simulink model "ASI_switch_Sami_FAHIM_R2022a"  (R2022a)
settings: Solver=VariableStepAuto  StartTime=0.0  StopTime=0.04  RelTol=1e-3
undefined symbols (not defined in the file): Az_I, Bz_I, Cz_I, Fz_I, Gz_I, Te, Vd
libraries: spsIGBTDiodeLib x4, cstblocks x4, spsSeriesRLCBranchLib x3, spsCurrentMeasurementLib x1, spsDCVoltageSourceLib x1, spsVoltageMeasurementLib x1, spspowerguiLib x1, simulink x1
settings Model: Creator=xshi  LastModifiedBy=sfahim

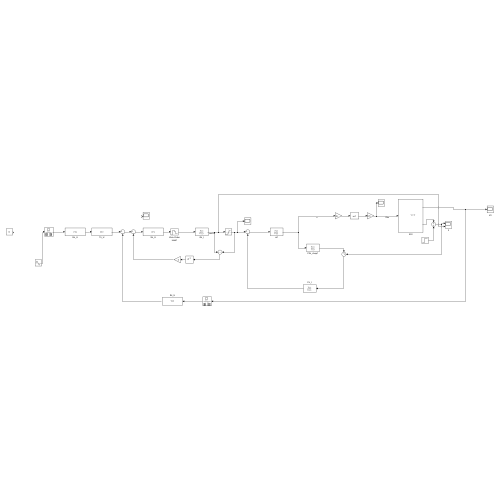
[thumbnail: Simulink's stored preview of the top-level diagram]
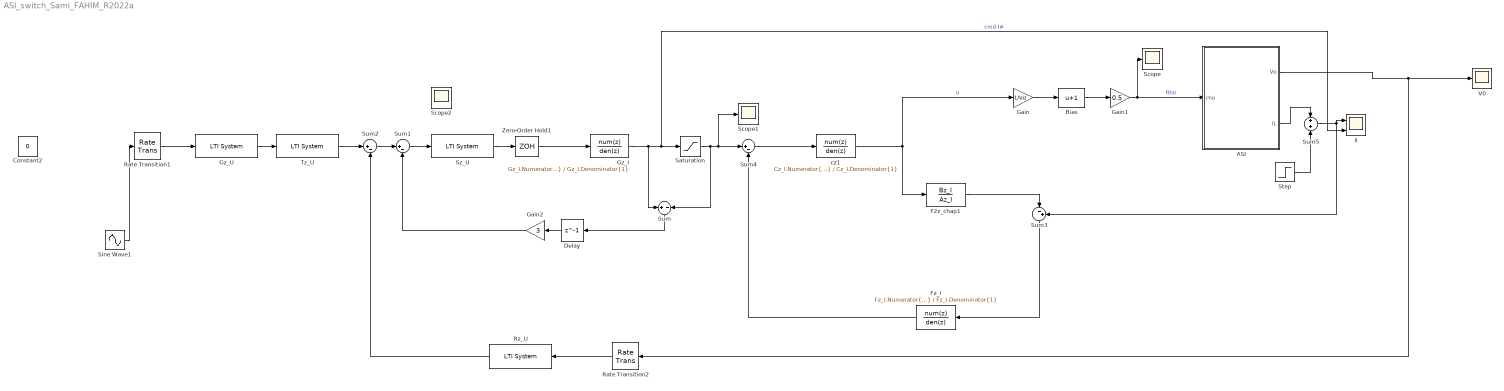
== system ASI_switch_Sami_FAHIM_R2022a ==
  ASI : Subsystem
      mask Display: image('C:\Users\xshi\Documents\Xuefang\Enseignement\4GE\COURS4GE\DS\DS 2024\Semestre 1\Matlab\ASI.png'); % Use "Edit Image" on toolstrip to change.
  Bias : Bias  Bias=1  SaturateOnIntegerOverflow=off
  Constant2 : Constant  Value=0  SampleTime=Te
  Delay : Delay  DelayLength=1
  F2z_chap1 : DiscreteTransferFcn  Numerator=Bz_I  Denominator=Az_I  SampleTime=Te
  Fz_I : DiscreteTransferFcn  Numerator=Fz_I.Numerator{1}  Denominator=Fz_I.Denominator{1}  SampleTime=Te
  Gain : Gain  Gain=1/Vd
  Gain1 : Gain  Gain=0.5
  Gain2 : Gain  Gain=3
  Gz_I : DiscreteTransferFcn  Numerator=Gz_I.Numerator{1}  Denominator=Gz_I.Denominator{1}  SampleTime=Te
  Gz_U : cstblocks/LTI System  sys=Gz_U  IC=[]
  Il : Scope  NumInputPorts=2
  Rate Transition1 : RateTransition  OutPortSampleTime=Te
  Rate Transition2 : RateTransition  OutPortSampleTime=Te
  Rz_U : cstblocks/LTI System  sys=Rz_U  IC=[]
  Saturation : Saturate  UpperLimit=25  LowerLimit=-25
  Scope : Scope
  Scope1 : Scope
  Scope2 : Scope
  Sine Wave1 : Sin  Amplitude=230  Frequency=314  SampleTime=0
  Step : Step  Time=0.01  After=0  SampleTime=0
  Sum : Sum  Inputs=+|-
  Sum1 : Sum  Inputs=|+-
  Sum2 : Sum  Inputs=|+-
  Sum3 : Sum  Inputs=|-+
  Sum4 : Sum  Inputs=|+-
  Sum5 : Sum  Inputs=+|+
  Sz_U : cstblocks/LTI System  sys=Sz_U  IC=[]
  Tz_U : cstblocks/LTI System  sys=Tz_U  IC=[]
  V0 : Scope
  Zero-Order Hold1 : ZeroOrderHold  SampleTime=Te
  cz1 : DiscreteTransferFcn  Numerator=Cz_I.Numerator{1}  Denominator=Cz_I.Denominator{1}  SampleTime=Te
  wires:
  Gain/1 -> Bias/1
  ASI/1(Vo) -> Rate Transition2/1, V0/1
  ASI/2(IL) -> Sum5/1
  Sz_U/1 -> Zero-Order Hold1/1
  Gz_U/1 -> Tz_U/1
  Rate Transition2/1 -> Rz_U/1
  Tz_U/1 -> Sum2/1
  Rz_U/1 -> Sum2/2
  Rate Transition1/1 -> Gz_U/1
  Sum3/1 -> Fz_I/1
  cz1/1 -> Gain/1, F2z_chap1/1  "u"
  Fz_I/1 -> Sum4/2
  Sum4/1 -> cz1/1
  Gz_I/1 -> Sum/1, Il/2, Saturation/1  "cmd I#"
  Zero-Order Hold1/1 -> Gz_I/1
  F2z_chap1/1 -> Sum3/1
  Bias/1 -> Gain1/1
  Gain1/1 -> Scope/1, ASI/1(rho)  "Rho"
  Sum/1 -> Delay/1
  Sum5/1 -> Sum3/2, Il/1
  Step/1 -> Sum5/2
  Delay/1 -> Gain2/1
  Saturation/1 -> Sum/2, Scope1/1, Sum4/1
  Sum2/1 -> Sum1/1
  Gain2/1 -> Sum1/2
  Sum1/1 -> Sz_U/1
  Sine Wave1/1 -> Rate Transition1/1

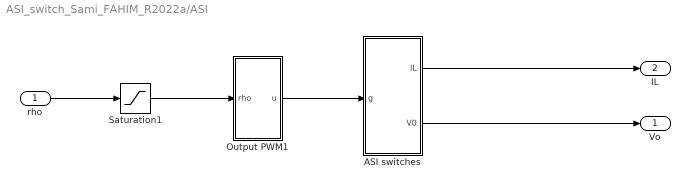
== system ASI_switch_Sami_FAHIM_R2022a/ASI ==
  rho : Inport
  ASI switches : Subsystem
  Output PWM1 : Subsystem
  Saturation1 : Saturate  UpperLimit=1  LowerLimit=0
  Vo : Outport  VectorParamsAs1DForOutWhenUnconnected=off
  IL : Outport  Port=2  VectorParamsAs1DForOutWhenUnconnected=off
  wires:
  Saturation1/1 -> Output PWM1/1(rho)
  rho/1 -> Saturation1/1
  Output PWM1/1(u) -> ASI switches/1(g)
  ASI switches/1(IL) -> IL/1
  ASI switches/2(V0) -> Vo/1

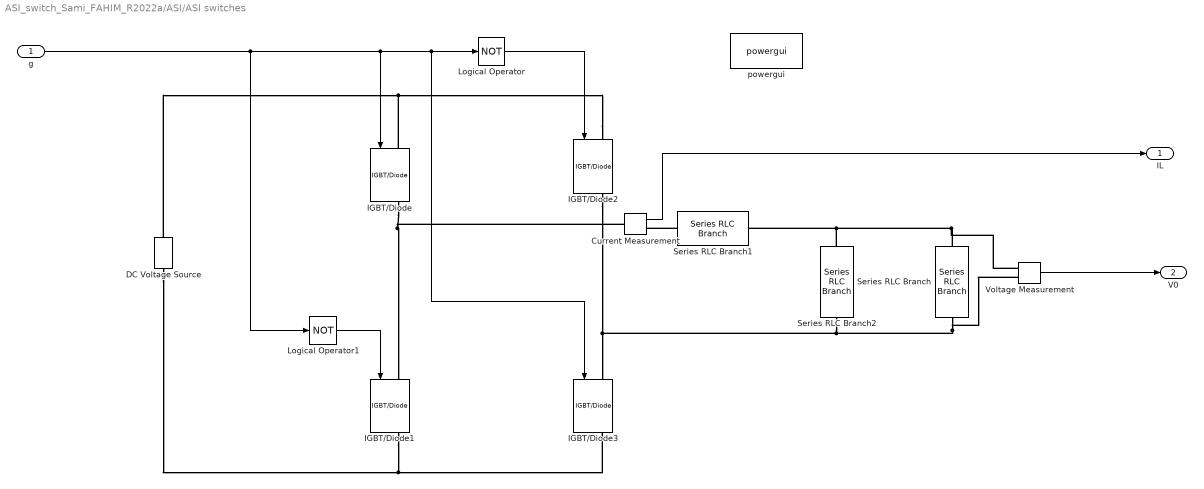
== system ASI_switch_Sami_FAHIM_R2022a/ASI/ASI switches ==
  g : Inport
  Current Measurement : spsCurrentMeasurementLib/Current Measurement  PhasorSimulation=off  OutputType=Complex  PSBequivalent=0
  DC Voltage Source : spsDCVoltageSourceLib/DC Voltage Source  Amplitude=250  Measurements=None
  IGBT/Diode{,1..3} (4 alike) : spsIGBTDiodeLib/IGBT//Diode  Ron=1e-3  Rs=1e5  Cs=inf  Measurements=on
  Logical Operator : Logic  Operator=NOT  AllPortsSameDT=off  OutDataTypeStr=boolean
  Logical Operator1 : Logic  Operator=NOT  AllPortsSameDT=off  OutDataTypeStr=boolean
  Series RLC Branch : spsSeriesRLCBranchLib/Series RLC Branch  LConnTagsString=__new0  RConnTagsString=__new0  BranchType=R  Resistance=10  Inductance=1e-3  SetiL0=off  InitialCurrent=0  Capacitance=1e-6  Setx0=off  InitialVoltage=0  Measurements=None
  Series RLC Branch1 : spsSeriesRLCBranchLib/Series RLC Branch  LConnTagsString=__new0  RConnTagsString=__new0  BranchType=RL  Resistance=0.195  Inductance=714e-6  SetiL0=off  InitialCurrent=0  Capacitance=1e-6  Setx0=off  InitialVoltage=0  Measurements=None
  Series RLC Branch2 : spsSeriesRLCBranchLib/Series RLC Branch  LConnTagsString=__new0  RConnTagsString=__new0  BranchType=RC  Resistance=0.07  Inductance=0  SetiL0=off  InitialCurrent=0  Capacitance=121.2e-6  Setx0=off  InitialVoltage=0  Measurements=None
  Voltage Measurement : spsVoltageMeasurementLib/Voltage Measurement  PhasorSimulation=off  OutputType=Complex  PSBequivalent=0
  powergui : spspowerguiLib/powergui  Priority=1  SimulationMode=Discrete  SampleTime=5.e-7  frequency=60  Iterations=50  frequencyindice=0  Pbase=100e6  ErrMax=1e-4  UnitsV=kV  UnitsW=MW  buscounter=0  FunctionMessages=off  echomessages=off  EnableUseOfTLC=off  CurrentSourceSwitches=off  DisableSnubberDevices=off  DisableRonSwitches=off  DisableVfSwitches=off  DisplayEquations=off  AutomaticDiscreteSolvers=off  SolverType=Tustin/Backward Euler (TBE)  Interpol=off  ExternalGateDelay=off  methode=off  Ts=100  x0status=blocks  SPID=on  SwTol=0  HookPort=off  NonlinearTolerance=1e-4  nMaxIteration=100  ContinueOnMaxIteration=off  RestoreLinks=warning  ResistiveCurrentMeasurement=off  Frange=[0:2:500]  Ylog=off  Xlog=on  ShowGrid=off  save=off  variable=ZData  structure=Vo  ZoomFFT=off  StartTime=0.01  cycles=1  DisplayStyle=1  fundamental=50  FreqAxis=off  MaxFrequency=1000  frequencyindicesteady=1  RmsSteady=1  display=off
  IL : Outport
  V0 : Outport  Port=2
  wires:
  Logical Operator/1 -> IGBT/Diode2/1
  g/1 -> Logical Operator1/1, IGBT/Diode3/1, Logical Operator/1, IGBT/Diode/1
  Logical Operator1/1 -> IGBT/Diode1/1
  Voltage Measurement/1 -> V0/1
  Current Measurement/1 -> IL/1
  connections:
  IGBT/Diode/RConn1 -- Current Measurement/LConn1 -- IGBT/Diode1/LConn1
  Series RLC Branch1/LConn1 -- Current Measurement/RConn1
  Series RLC Branch/RConn1 -- Series RLC Branch2/RConn1 -- IGBT/Diode2/RConn1 -- IGBT/Diode3/LConn1 -- Voltage Measurement/LConn2
  DC Voltage Source/LConn1 -- IGBT/Diode1/RConn1 -- IGBT/Diode3/RConn1
  Series RLC Branch/LConn1 -- Voltage Measurement/LConn1 -- Series RLC Branch2/LConn1 -- Series RLC Branch1/RConn1
  IGBT/Diode2/LConn1 -- DC Voltage Source/RConn1 -- IGBT/Diode/LConn1

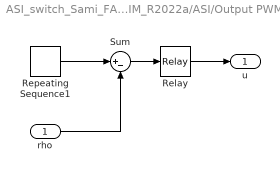
== system ASI_switch_Sami_FAHIM_R2022a/ASI/Output PWM1 ==
  rho : Inport
  Relay : Relay  OnSwitchValue=0  OffSwitchValue=0  OnOutputValue=0  OffOutputValue=1
  Repeating Sequence1 : simulink/Sources/Repeating Sequence  rep_seq_t=[0 Te]  rep_seq_y=[0 1]
  Sum : Sum  Inputs=|+-  SaturateOnIntegerOverflow=on
  u : Outport  VectorParamsAs1DForOutWhenUnconnected=off
  wires:
  Repeating Sequence1/1 -> Sum/1
  rho/1 -> Sum/2
  Sum/1 -> Relay/1
  Relay/1 -> u/1
